simulink model "AUT580_Joystick_communication"  (R2023a)
settings: Solver=FixedStepDiscrete  StartTime=0.0  StopTime=inf  FixedStep=0.004  RelTol=1e-3
undefined symbols (not defined in the file or in its folder): f, Joystick, Standard_Devices, UDP_Protocol
libraries: sldrtlib x4, aerolibanimutils x1, instrumentlib x1
settings Model: Creator=mustalah  LastModifiedBy=mustalah
settings DebuggingCC: UnconnectedInputMsg=warning  UnconnectedOutputMsg=warning  UnconnectedLineMsg=warning
settings ModelReferenceCC: EnableRefExpFcnMdlSchedulingChecks=on
settings RTWCC: DLArmComputeVersion=19.05

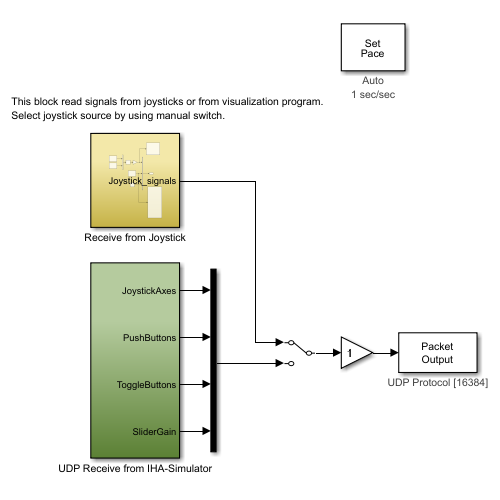
[thumbnail: Simulink's stored preview of the top-level diagram]
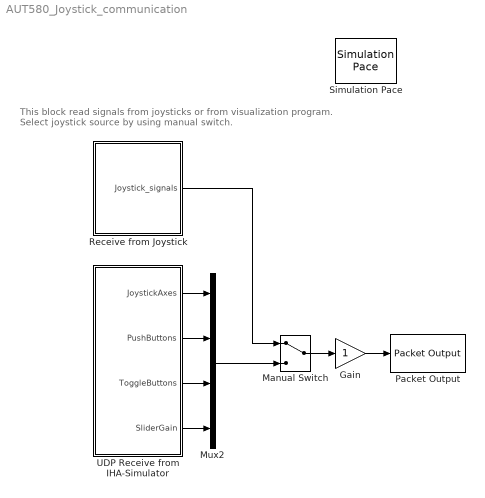
== system AUT580_Joystick_communication ==
  note: This block read signals from joysticks or from visualization program.
      | Select joystick source by using manual switch.
  Gain : Gain
  Manual Switch : ManualSwitch
  Mux2 : Mux
  Packet Output : sldrtlib/Packet Output  SampleTime=0.012  MaxMissedTicks=1000  ShowMissedTicks=off  YieldWhenWaiting=off  DrvName=Standard_Devices/UDP_Protocol  DrvAddress=16384  DrvOptions=[0 8052 49 57 50 46 49 54 56 46 49 48 46 50 0 0 0 0 0 0 0 0 0 0 0 0 0 0 0 0 0 0 0 0 0 0 0 0 0 0 0 0 0 0 0 0 0 0 0 0 0 0 0 0 0 0 0 0 0 0 0 0 0 0 0 0 0 0 0 0 0 0 0 0 0 0 0 0 0 0 0 0 0 0 0 0 0 0 0 0 0 0 0 0 0 0 0 0 0 0 0 0 0 0 0 0 0 0 0 0 0 0 0 0 0 0 0 0 0 0 0 0 0 0 0 0 0 0 0 0 0 0 0 0 0 0 0 0 0 0 0 0 0 0 0 0 0 0 0 0 0 0 0 0 0 0 0 0 0 0 0 0 0 0 0 0 0 0 0 0 0 0 0 0 0 0 0 0 0 0 0 0 0 0 0 0 0 0 0 0 0 0 0 0 0 0 0 0 0 0 0 0 0 0 0 0 0 0 0 0 0 0 0 0 0 0 0 0 0 0 0 0 0 0 0 0 0 0 0 0 0 0 0 0 0 0 0 0 0 0 0 0 0 0 0 0 0 0 0 0 0 0 0 0 0 0]  PacketSize=152  DataTypes={'19*double'}  ShowReady=off  ShowError=off  PacketID=1  ByteOrder=1  InitialValue=[]  FinalValue=[]
      settings: AttributesFormatString=UDP Protocol [16384]
  Receive from Joystick : Subsystem
  Simulation Pace : aerolibanimutils/Simulation Pace  SimulationPace=1  SleepMode=Auto  OutputPaceError=off  SampleTime=0.012
  UDP Receive from IHA-Simulator : Subsystem
  wires:
  UDP Receive from IHA-Simulator/1(JoystickAxes) -> Mux2/1
  UDP Receive from IHA-Simulator/2(PushButtons) -> Mux2/2
  UDP Receive from IHA-Simulator/3(ToggleButtons) -> Mux2/3
  UDP Receive from IHA-Simulator/4(SliderGain) -> Mux2/4
  Gain/1 -> Packet Output/1
  Manual Switch/1 -> Gain/1
  Mux2/1 -> Manual Switch/2
  Receive from Joystick/1(Joystick_signals) -> Manual Switch/1

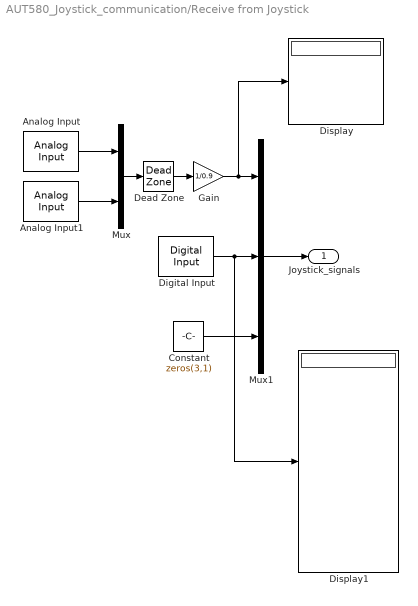
== system AUT580_Joystick_communication/Receive from Joystick ==
  Analog Input : sldrtlib/Analog Input  SampleTime=0.012  MaxMissedTicks=1000  ShowMissedTicks=off  YieldWhenWaiting=off  DrvName=Standard_Devices/Joystick  DrvAddress=1  DrvOptions=zeros(1,0)  Channels=[1:2]  RangeMode=2  VoltRange=1  DataType=1
      settings: AttributesFormatString=Joystick [1]
  Analog Input1 : sldrtlib/Analog Input  SampleTime=0.012  MaxMissedTicks=1000  ShowMissedTicks=off  YieldWhenWaiting=off  DrvName=Standard_Devices/Joystick  DrvAddress=2  DrvOptions=zeros(1,0)  Channels=[1:2]  RangeMode=2  VoltRange=1  DataType=1
      settings: AttributesFormatString=Joystick [2]
  Constant : Constant  Value=zeros(3,1)  OutDataTypeStr=double
  Dead Zone : DeadZone  LowerValue=-0.1  UpperValue=0.1
  Digital Input : sldrtlib/Digital Input  SampleTime=0.012  MaxMissedTicks=1000  ShowMissedTicks=off  YieldWhenWaiting=off  DrvName=Standard_Devices/Joystick  DrvAddress=1  DrvOptions=zeros(1,0)  Channels=[1:12]  BitMode=1  DataType=1
      settings: AttributesFormatString=Joystick [1]
  Display : Display
  Display1 : Display
  Gain : Gain  Gain=1/0.9
  Mux : Mux  Inputs=2
  Mux1 : Mux  Inputs=3
  Joystick_signals : Outport  OutDataTypeStr=double  PortDimensions=19
  wires:
  Analog Input/1 -> Mux/1
  Gain/1 -> Display/1, Mux1/1
  Mux1/1 -> Joystick_signals/1
  Dead Zone/1 -> Gain/1
  Analog Input1/1 -> Mux/2
  Constant/1 -> Mux1/3
  Mux/1 -> Dead Zone/1
  Digital Input/1 -> Display1/1, Mux1/2

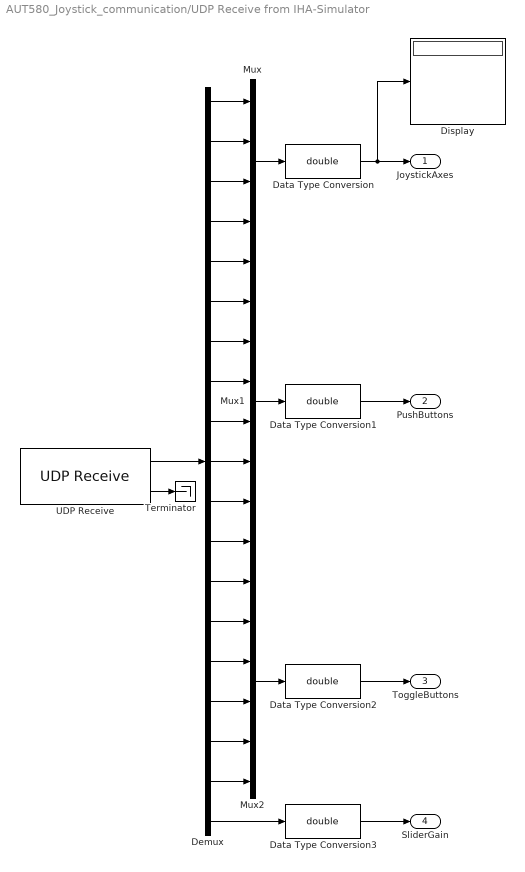
== system AUT580_Joystick_communication/UDP Receive from IHA-Simulator ==
  Data Type Conversion{,1..3} (4 alike) : DataTypeConversion  OutDataTypeStr=double  SaturateOnIntegerOverflow=off  RndMeth=Floor
  Demux : Demux  Outputs=19
  Display : Display
  Mux : Mux
  Mux1 : Mux  Inputs=8
  Mux2 : Mux  Inputs=6
  Terminator : Terminator
  UDP Receive : instrumentlib/UDP Receive  Host=localhost  Port=9090  LocalPort=8051  EnablePortSharing=off  GetLatestData=off  DataSize=19  DataType=single  ASCIIFormatting=%f,  Terminator=LF  ByteOrder=LittleEndian  EnableBlockingMode=off  Timeout=10  SampleTime=4e-3  LocalAddress=127.0.0.1
  JoystickAxes : Outport
  PushButtons : Outport  Port=2
  ToggleButtons : Outport  Port=3
  SliderGain : Outport  Port=4
  wires:
  UDP Receive/1 -> Demux/1
  UDP Receive/2 -> Terminator/1
  Mux/1 -> Data Type Conversion/1
  Demux/1 -> Mux/1
  Demux/2 -> Mux/2
  Demux/3 -> Mux/3
  Demux/4 -> Mux/4
  Demux/5 -> Mux1/1
  Demux/6 -> Mux1/2
  Demux/7 -> Mux1/3
  Demux/8 -> Mux1/4
  Demux/9 -> Mux1/5
  Demux/10 -> Mux1/6
  Demux/11 -> Mux1/7
  Mux1/1 -> Data Type Conversion1/1
  Demux/12 -> Mux1/8
  Demux/13 -> Mux2/1
  Demux/14 -> Mux2/2
  Demux/15 -> Mux2/3
  Demux/16 -> Mux2/4
  Demux/17 -> Mux2/5
  Demux/18 -> Mux2/6
  Mux2/1 -> Data Type Conversion2/1
  Demux/19 -> Data Type Conversion3/1
  Data Type Conversion/1 -> Display/1, JoystickAxes/1
  Data Type Conversion1/1 -> PushButtons/1
  Data Type Conversion2/1 -> ToggleButtons/1
  Data Type Conversion3/1 -> SliderGain/1
